simulink model "modello2"  (R2019a)
settings: Solver=VariableStepAuto  StartTime=0.0  StopTime=10.0  RelTol=1e-3
libraries: simulink x3, shared6dof x1, simulink_extras x1
settings Model: Creator=edoardo  LastModifiedBy=edoardo

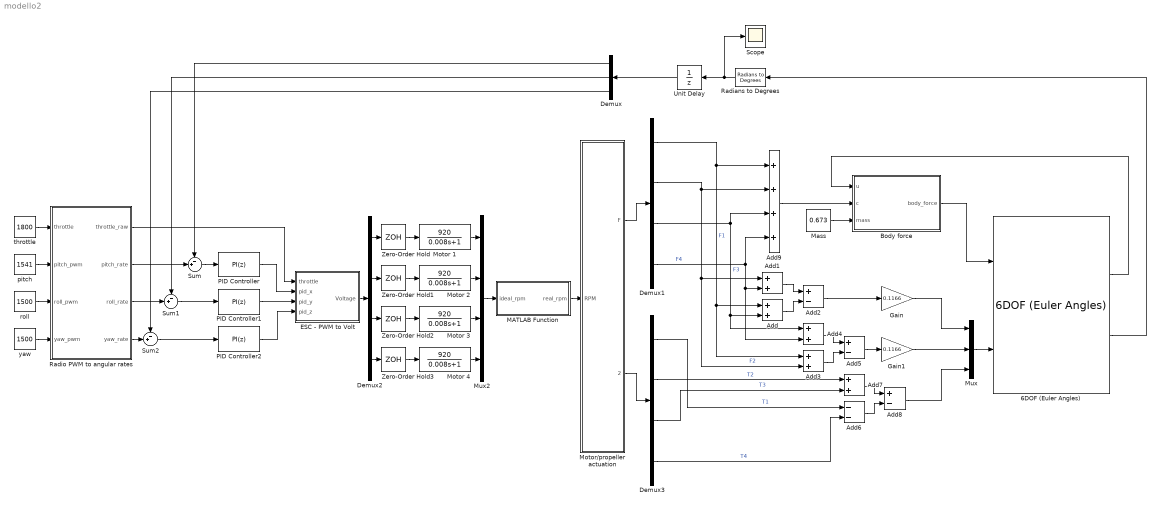
== system modello2 ==
  6DOF (Euler Angles) : shared6dof/6DOF (Euler Angles)  units=Metric (MKS)  mtype=Fixed  rep=Euler Angles  xme_0=[0 0 0]  Vm_0=[0 0 0]  eul_0=[0 0 0]  pm_0=[0 0 0]  mass_0=0.673  mass_e=0.5  mass_f=2.0  inertia=[0.00305 0 0; 0 0.00305 0; 0 0 0.00611]  inertia_e=eye(3)  inertia_f=2*eye(3)  k_quat=1.0  vre_flag=on  abi_flag=off  aMode=0  xme_statename=''  Vm_statename=''  eul_statename=''  quat_statename=''  pm_statename=''  mass_statename=''
      settings: SourceProductBaseCode=AE
  Add{,1,3..4,7} (5 alike) : Sum
  Add2 : Sum  Inputs=+-
  Add5 : Sum  Inputs=+-
  Add6 : Sum  Inputs=--
  Add8 : Sum  Inputs=+-
  Add9 : Sum  Inputs=++++
  Body force : MATLAB Function  TreatAsAtomicUnit=on
  Demux : Demux  Outputs=3
  Demux1 : Demux
  Demux2 : Demux
  Demux3 : Demux
  "ESC - PWM to Volt " : MATLAB Function  TreatAsAtomicUnit=on
  Gain : Gain  Gain=0.1166
  Gain1 : Gain  Gain=0.1166
  MATLAB Function : MATLAB Function  TreatAsAtomicUnit=on
  Mass : Constant  Value=0.673
  Motor {1..4} (4 alike) : TransferFcn  Numerator=[920]  Denominator=[0.008 1]
  Motor/propeller actuation : MATLAB Function  TreatAsAtomicUnit=on
  Mux : Mux  Inputs=3
  Mux2 : Mux
  PID Controller : simulink/Continuous/PID Controller  Controller=PI  Form=Parallel  TimeDomain=Discrete-time  SampleTime=0.002041  IntegratorMethod=Backward Euler  FilterMethod=Backward Euler  ControllerParametersSource=internal  P=1.1  I=0.002  D=0.002  UseFilter=off  N=100  TunerSelectOption=Transfer Function Based (PID Tuner App)  InitialConditionSource=internal  InitialConditionForIntegrator=0  InitialConditionForFilter=0  DifferentiatorICPrevScaledInput=0  ExternalReset=none  TrackingMode=off  Kt=1  LimitOutput=on  UpperSaturationLimit=400  LowerSaturationLimit=-400  LinearizeAsGain=off  AntiWindupMode=clamping  Kb=1  POutMin=[]  POutMax=[]  IOutMin=[]  IOutMax=[]  DOutMin=[]  DOutMax=[]  NOutMin=[]  NOutMax=[]  SumOutMin=[]  SumOutMax=[]  SaturationOutMin=[]  SaturationOutMax=[]  PParamMin=[]  PParamMax=[]  IParamMin=[]  IParamMax=[]  DParamMin=[]  DParamMax=[]  NParamMin=[]  NParamMax=[]  KbParamMin=[]  KbParamMax=[]  KtParamMin=[]  KtParamMax=[]  KbOutMin=[]  KbOutMax=[]  KtOutMin=[]  KtOutMax=[]  IntegratorOutMin=[]  IntegratorOutMax=[]  FilterOutMin=[]  FilterOutMax=[]  SumI1OutMin=[]  SumI1OutMax=[]  SumI2OutMin=[]  SumI2OutMax=[]  SumI3OutMin=[]  SumI3OutMax=[]  SumI4OutMin=[]  SumI4OutMax=[]  SumDOutMin=[]  SumDOutMax=[]  DifferentiatorOutMin=[]  DifferentiatorOutMax=[]  FilterDiffOutCoefMin=[]  FilterDiffOutCoefMax=[]  ReciprocalOutMin=[]  ReciprocalOutMax=[]  SumDenOutMin=[]  SumDenOutMax=[]  SumNumOutMin=[]  SumNumOutMax=[]  DivideOutMin=[]  DivideOutMax=[]  IntegratorContinuousStateAttributes=''  IntegratorStateMustResolveToSignalObject=off  IntegratorRTWStateStorageClass=Auto  FilterContinuousStateAttributes=''  FilterStateMustResolveToSignalObject=off  FilterRTWStateStorageClass=Auto  ParallelPVariant=InternalParameters  IdealPVariant=Disabled  IVariant=InternalParameters  DVariant=Disabled  IntegratorVariant=Discrete  SatVariant=Enabled  AWVariant=DiscClampingParallel  PCopyVariant=Disabled  TRVariant=Disabled  FdbkBlocksVariant=Feedback  IdealPFdbkVariant=Passthrough  SatFdbkVariant=Passthrough  DerivativeFilterVariant=Disabled  NVariant=Disabled  NCopyVariant=Disabled_SignalSpec  FilterICVariant=Disabled  IntegratorICVariant=InternalICs  ExternalResetVariant=Disabled  TRSumVariant=Passthrough  SumFdbkVariant=Enabled  SumVariant=Sum_PI
  PID Controller1 : simulink/Continuous/PID Controller  Controller=PI  Form=Parallel  TimeDomain=Discrete-time  SampleTime=0.002041  IntegratorMethod=Backward Euler  FilterMethod=Backward Euler  ControllerParametersSource=internal  P=1.1  I=0.02  D=0.005  UseFilter=off  N=37.6645512562197  TunerSelectOption=Transfer Function Based (PID Tuner App)  InitialConditionSource=internal  InitialConditionForIntegrator=0  InitialConditionForFilter=0  DifferentiatorICPrevScaledInput=0  ExternalReset=none  TrackingMode=off  Kt=1  LimitOutput=on  UpperSaturationLimit=400  LowerSaturationLimit=-400  LinearizeAsGain=off  AntiWindupMode=clamping  Kb=1  POutMin=[]  POutMax=[]  IOutMin=[]  IOutMax=[]  DOutMin=[]  DOutMax=[]  NOutMin=[]  NOutMax=[]  SumOutMin=[]  SumOutMax=[]  SaturationOutMin=[]  SaturationOutMax=[]  PParamMin=[]  PParamMax=[]  IParamMin=[]  IParamMax=[]  DParamMin=[]  DParamMax=[]  NParamMin=[]  NParamMax=[]  KbParamMin=[]  KbParamMax=[]  KtParamMin=[]  KtParamMax=[]  KbOutMin=[]  KbOutMax=[]  KtOutMin=[]  KtOutMax=[]  IntegratorOutMin=[]  IntegratorOutMax=[]  FilterOutMin=[]  FilterOutMax=[]  SumI1OutMin=[]  SumI1OutMax=[]  SumI2OutMin=[]  SumI2OutMax=[]  SumI3OutMin=[]  SumI3OutMax=[]  SumI4OutMin=[]  SumI4OutMax=[]  SumDOutMin=[]  SumDOutMax=[]  DifferentiatorOutMin=[]  DifferentiatorOutMax=[]  FilterDiffOutCoefMin=[]  FilterDiffOutCoefMax=[]  ReciprocalOutMin=[]  ReciprocalOutMax=[]  SumDenOutMin=[]  SumDenOutMax=[]  SumNumOutMin=[]  SumNumOutMax=[]  DivideOutMin=[]  DivideOutMax=[]  IntegratorContinuousStateAttributes=''  IntegratorStateMustResolveToSignalObject=off  IntegratorRTWStateStorageClass=Auto  FilterContinuousStateAttributes=''  FilterStateMustResolveToSignalObject=off  FilterRTWStateStorageClass=Auto  ParallelPVariant=InternalParameters  IdealPVariant=Disabled  IVariant=InternalParameters  DVariant=Disabled  IntegratorVariant=Discrete  SatVariant=Enabled  AWVariant=DiscClampingParallel  PCopyVariant=Disabled  TRVariant=Disabled  FdbkBlocksVariant=Feedback  IdealPFdbkVariant=Passthrough  SatFdbkVariant=Passthrough  DerivativeFilterVariant=Disabled  NVariant=Disabled  NCopyVariant=Disabled_SignalSpec  FilterICVariant=Disabled  IntegratorICVariant=InternalICs  ExternalResetVariant=Disabled  TRSumVariant=Passthrough  SumFdbkVariant=Enabled  SumVariant=Sum_PI
  PID Controller2 : simulink/Continuous/PID Controller  Controller=PI  Form=Parallel  TimeDomain=Discrete-time  SampleTime=0.002041  IntegratorMethod=Backward Euler  FilterMethod=Backward Euler  ControllerParametersSource=internal  P=4  I=0.02  D=0.003  UseFilter=off  N=100  TunerSelectOption=Transfer Function Based (PID Tuner App)  InitialConditionSource=internal  InitialConditionForIntegrator=0  InitialConditionForFilter=0  DifferentiatorICPrevScaledInput=0  ExternalReset=none  TrackingMode=off  Kt=1  LimitOutput=on  UpperSaturationLimit=400  LowerSaturationLimit=-400  LinearizeAsGain=off  AntiWindupMode=clamping  Kb=1  POutMin=[]  POutMax=[]  IOutMin=[]  IOutMax=[]  DOutMin=[]  DOutMax=[]  NOutMin=[]  NOutMax=[]  SumOutMin=[]  SumOutMax=[]  SaturationOutMin=[]  SaturationOutMax=[]  PParamMin=[]  PParamMax=[]  IParamMin=[]  IParamMax=[]  DParamMin=[]  DParamMax=[]  NParamMin=[]  NParamMax=[]  KbParamMin=[]  KbParamMax=[]  KtParamMin=[]  KtParamMax=[]  KbOutMin=[]  KbOutMax=[]  KtOutMin=[]  KtOutMax=[]  IntegratorOutMin=[]  IntegratorOutMax=[]  FilterOutMin=[]  FilterOutMax=[]  SumI1OutMin=[]  SumI1OutMax=[]  SumI2OutMin=[]  SumI2OutMax=[]  SumI3OutMin=[]  SumI3OutMax=[]  SumI4OutMin=[]  SumI4OutMax=[]  SumDOutMin=[]  SumDOutMax=[]  DifferentiatorOutMin=[]  DifferentiatorOutMax=[]  FilterDiffOutCoefMin=[]  FilterDiffOutCoefMax=[]  ReciprocalOutMin=[]  ReciprocalOutMax=[]  SumDenOutMin=[]  SumDenOutMax=[]  SumNumOutMin=[]  SumNumOutMax=[]  DivideOutMin=[]  DivideOutMax=[]  IntegratorContinuousStateAttributes=''  IntegratorStateMustResolveToSignalObject=off  IntegratorRTWStateStorageClass=Auto  FilterContinuousStateAttributes=''  FilterStateMustResolveToSignalObject=off  FilterRTWStateStorageClass=Auto  ParallelPVariant=InternalParameters  IdealPVariant=Disabled  IVariant=InternalParameters  DVariant=Disabled  IntegratorVariant=Discrete  SatVariant=Enabled  AWVariant=DiscClampingParallel  PCopyVariant=Disabled  TRVariant=Disabled  FdbkBlocksVariant=Feedback  IdealPFdbkVariant=Passthrough  SatFdbkVariant=Passthrough  DerivativeFilterVariant=Disabled  NVariant=Disabled  NCopyVariant=Disabled_SignalSpec  FilterICVariant=Disabled  IntegratorICVariant=InternalICs  ExternalResetVariant=Disabled  TRSumVariant=Passthrough  SumFdbkVariant=Enabled  SumVariant=Sum_PI
  Radians to Degrees : simulink_extras/Transformations/Radians to Degrees
  Radio PWM to angular rates : MATLAB Function  TreatAsAtomicUnit=on
  Scope : Scope
  Sum : Sum  Inputs=-+|
  Sum1 : Sum  Inputs=-+|
  Sum2 : Sum  Inputs=-+|
  Unit Delay : UnitDelay  SampleTime=-1  HasFrameUpgradeWarning=on
  Zero-Order Hold{,1..3} (4 alike) : ZeroOrderHold  SampleTime=-1
  pitch : Constant  Value=1541
  roll : Constant  Value=1500
  throttle : Constant  Value=1800
  yaw : Constant  Value=1500
  wires:
  yaw/1 -> Radio PWM to angular rates/4(yaw_pwm)
  roll/1 -> Radio PWM to angular rates/3(roll_pwm)
  pitch/1 -> Radio PWM to angular rates/2(pitch_pwm)
  throttle/1 -> Radio PWM to angular rates/1(throttle)
  Demux/2 -> Sum1/1
  Demux/1 -> Sum/1
  Sum/1 -> PID Controller/1
  Radio PWM to angular rates/2(pitch_rate) -> Sum/2
  PID Controller/1 -> "ESC - PWM to Volt "/2(pid_x)
  Demux/3 -> Sum2/1
  PID Controller2/1 -> "ESC - PWM to Volt "/4(pid_z)
  Sum2/1 -> PID Controller2/1
  PID Controller1/1 -> "ESC - PWM to Volt "/3(pid_y)
  Sum1/1 -> PID Controller1/1
  Unit Delay/1 -> Demux/1
  6DOF (Euler Angles)/6 -> Radians to Degrees/1
  Demux2/4 -> Zero-Order Hold3/1
  Demux2/1 -> Zero-Order Hold/1
  Zero-Order Hold1/1 -> Motor 2/1
  Demux2/3 -> Zero-Order Hold2/1
  Demux2/2 -> Zero-Order Hold1/1
  "ESC - PWM to Volt "/1(Voltage) -> Demux2/1
  Motor 3/1 -> Mux2/3
  Zero-Order Hold/1 -> Motor 1/1
  Zero-Order Hold2/1 -> Motor 3/1
  Motor 1/1 -> Mux2/1
  Motor 4/1 -> Mux2/4
  Motor 2/1 -> Mux2/2
  Zero-Order Hold3/1 -> Motor 4/1
  Radio PWM to angular rates/3(roll_rate) -> Sum1/2
  Radio PWM to angular rates/4(yaw_rate) -> Sum2/2
  Radio PWM to angular rates/1(throttle_raw) -> "ESC - PWM to Volt "/1(throttle)
  Mux2/1 -> MATLAB Function/1(ideal_rpm)
  MATLAB Function/1(real_rpm) -> Motor/propeller actuation/1(RPM)
  Radians to Degrees/1 -> Scope/1, Unit Delay/1
  Motor/propeller actuation/1(F) -> Demux1/1
  Demux1/1 -> Add9/1, Add3/1, Add/1  "F1"
  Demux1/3 -> Add9/3, Add4/1, Add/2  "F3"
  Demux1/2 -> Add9/2, Add3/2, Add1/1  "F2"
  Demux1/4 -> Add9/4, Add4/2, Add1/2  "F4"
  Add1/1 -> Add2/1
  Add/1 -> Add2/2
  Add4/1 -> Add5/1
  Add3/1 -> Add5/2
  Add6/1 -> Add8/2
  Add7/1 -> Add8/1
  Add2/1 -> Gain/1
  Add5/1 -> Gain1/1
  Gain/1 -> Mux/1
  Gain1/1 -> Mux/2
  Add8/1 -> Mux/3
  Motor/propeller actuation/2(Torque) -> Demux3/1
  Demux3/2 -> Add7/1  "T2"
  Demux3/3 -> Add7/2  "T3"
  Demux3/1 -> Add6/1  "T1"
  Demux3/4 -> Add6/2  "T4"
  Mux/1 -> 6DOF (Euler Angles)/2
  Mass/1 -> Body force/3(mass)
  Add9/1 -> Body force/2(c)
  6DOF (Euler Angles)/3 -> Body force/1(u)
  Body force/1(body_force) -> 6DOF (Euler Angles)/1

== matlab function modello2/Body force ==
  data: u input; body_force output; c input; mass input
function body_force = fcn(u,c,mass)

    %gli angoli che mi porto dalla retroazione
    phi   = u(1);
    theta = u(2);
    psi   = u(3);
    
    %le matrici di rotazione che mi servono per le accelerazioni
    Rx = [     1        0           0 
               0      cos(phi)   -sin(phi)
               0      sin(phi)    cos(phi) ];
       
    
    Ry = [ cos(theta)    0       sin(theta)
               0         1          0
          -sin(theta)    0       cos(theta) ];
      
      
    Rz = [ cos(psi)  -sin(psi)      0
           sin(psi)   cos(psi)      0
               0         0          1 ];
    %la rotazione è uguale al prodotto delle matrici di rotazione valutate negli angoli       
    R = Rz*Ry*Rx;
    %il vettore delle forze del corpo è calcolato come segue e riportato
    %come output
    body_force = mass * [0; 0; 9.81] - R * [0; 0; c];
    
end

== matlab function modello2/ESC - PWM to Volt  ==
  data: throttle input; pid_x input; Voltage output; pid_y input; pid_z input

function Voltage = fcn(throttle,pid_x,pid_y,pid_z)
    %Parameters names, except the phisical ones, are directly taken from the C code implementation i.o.t. have 1:1 match  
    Voltage        = [0;0;0;0];
    
    if( throttle > 1800 )
        throttle = 1800;  %leave room for PID controller
    end
    
    Voltage(1) = throttle-pid_y-pid_x-pid_z;  %rear  right motor PWM
    Voltage(2) = throttle-pid_y+pid_x+pid_z;  %front right motor PWM
    Voltage(3) = throttle+pid_y-pid_x+pid_z;  %rear   left motor PWM
	Voltage(4) = throttle+pid_y+pid_x-pid_z;  %front  left motor PWM
   
    
    for i = 1:4  
        if( Voltage(i) > 2000 )
            Voltage(i) = 2000;
        end
        
        if( Voltage(i) < 1100 )
            Voltage(i) = 1100;
        end
        
        Voltage(i) = (Voltage(i)-1000)*0.0111;
    end

end

== matlab function modello2/Radio PWM to angular rates ==
  data: throttle input; throttle_raw output; pitch_pwm input; roll_pwm input; yaw_pwm input; pitch_rate output; roll_rate output; yaw_rate output
function [throttle_raw,pitch_rate,roll_rate,yaw_rate] = fcn(throttle,pitch_pwm,roll_pwm,yaw_pwm)

DEADBAND_UPPER_BOUND      = 1508;
DEADBAND_LOWER_BOUND      = 1492;
SETPOINT_PITCH_SPEED_RATE = 3.0;
SETPOINT_ROLL_SPEED_RATE  = 3.0;
SETPOINT_YAW_SPEED_RATE   = 3.0;

pitch_rate   = 0;
roll_rate    = 0;
yaw_rate     = 0;
throttle_raw = throttle;

if( pitch_pwm > DEADBAND_UPPER_BOUND )
    pitch_rate = ( pitch_pwm - DEADBAND_UPPER_BOUND ) / SETPOINT_PITCH_SPEED_RATE;
end
if( pitch_pwm < DEADBAND_LOWER_BOUND )
    pitch_rate = ( pitch_pwm - DEADBAND_LOWER_BOUND ) / SETPOINT_PITCH_SPEED_RATE;
end

if( roll_pwm > DEADBAND_UPPER_BOUND )
    roll_rate = ( roll_pwm - DEADBAND_UPPER_BOUND ) / SETPOINT_ROLL_SPEED_RATE;
end
if( roll_pwm < DEADBAND_LOWER_BOUND )
    roll_rate = ( roll_pwm - DEADBAND_LOWER_BOUND ) / SETPOINT_ROLL_SPEED_RATE;
end

if( yaw_pwm > DEADBAND_UPPER_BOUND )
    yaw_rate = ( yaw_pwm - DEADBAND_UPPER_BOUND ) / SETPOINT_YAW_SPEED_RATE;
end
if( yaw_pwm < DEADBAND_LOWER_BOUND )
    yaw_rate = ( yaw_pwm - DEADBAND_LOWER_BOUND ) / SETPOINT_YAW_SPEED_RATE;
end

end

== matlab function modello2/Motor//propeller actuation ==
  data: F output; RPM input; Torque output
function [F,Torque]  = fcn(RPM)
    
    Torque = [0 0 0 0];
    F      = [0 0 0 0];

    for i = 1:4
        Ct         = 6.3*10^-19*RPM(i)^4-1.51*10^-14*RPM(i)^3+1.21*10^-10*RPM(i)^2-2.58*10^-7*RPM(i)+0.12;
        F(i)       = Ct*1.225*(RPM(i)/60)^2*0.001704;
        Torque(i)  = -1.79*10^-26*RPM(i)^6+4.63*10^-21*RPM(i)^5-1.37*10^-16*RPM(i)^4+1.5*10^-12*RPM(i)^3-5.96*10^-9*RPM(i)^2+1.11*10^-5*RPM(i)+4.52*10^-4;     
    end
    
end

== matlab function modello2/MATLAB Function ==
  data: ideal_rpm input; real_rpm output
function real_rpm = fcn(ideal_rpm)

    real_rpm = [0 0 0 0];
    
    for i = 1:4
        real_rpm(i) = -2.4*10^-9*ideal_rpm(i)^3-9.22*10^-21*ideal_rpm(i)^2+ideal_rpm(i)+9.36*10^-15;
    end

end
